simulink model "MFunction"  (Simulink 7.5)
settings: Solver=ode45  StartTime=0.0  StopTime=5  RelTol=1e-3
settings Model: Creator=Simon  LastModifiedBy=Simon

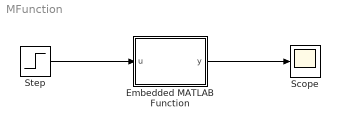
== system MFunction ==
  Embedded MATLAB Function : Stateflow chart  TreatAsAtomicUnit=on
  Scope : Scope
  Step : Step  SampleTime=0
  wires:
  Step/1 -> Embedded MATLAB Function/1(u)
  Embedded MATLAB Function/1(y) -> Scope/1

== matlab function Embedded MATLAB Function ==
  data: u input double; y output double
function y = fcn(u)
%#eml

y = 2*u;
